simulink model "Simulator_Part_12"  (R2019b)
settings: Solver=FixedStepAuto  StartTime=0.0  StopTime=tfinal  FixedStep=dt  RelTol=1e-3
model workspace (MAT data in the model file):
  s000 = 0
values from neighbouring files (symbols this model uses):
  dc = [ aircraft_data(57:59) * pi/180 ; aircraft_data(60)]    [Aircraft_Simulator.m]    (also in Plot1.m = [da 0 0 0]; Plot2.m = [0 0 0 dT]; Plot3.m = [0 0 0 dT]; Plot4.m = [0 0 0 dT])
  Fg_0 = m*g*[sin(s0(8)); -cos(s0(8))*sin(s0(7)); -cos(s0(8))*cos(s0(7))]    [Aircraft_Simulator.m]
  g = aircraft_data(52)    [Aircraft_Simulator.m]    (also in Airframe_Model.m = 32.17405)
  Ixx = aircraft_data(53)    [Aircraft_Simulator.m]    (also in Airframe_Model.m = I(1))
  Iyy = aircraft_data(54)    [Aircraft_Simulator.m]    (also in Airframe_Model.m = I(5))
  Izz = aircraft_data(55)    [Aircraft_Simulator.m]    (also in Airframe_Model.m = I(9))
  K = struct('u',s0(1),'v',s0(2),'w',s0(3),'p',s0(4),'q',s0(5),     'r',s0(6),'phi',s0(7),'theta',s0(8),'psi',s0(9),'x',s0(10),     'y',s0(11),'z',s0(12),'alpha',s0(8),'beta',0,'V_t',Vto,'w_dot',0)    [Aircraft_Simulator.m]
  m = aircraft_data(51)    [Aircraft_Simulator.m]
  M_0 = [0; 0; 0]    [Aircraft_Simulator.m]
  Matrix_Controllers = [0     0       Xde   Xdth ... (first row only)    [Aircraft_Simulator.m]
  Matrix_states = [Xu   0   Xw   0   0   0   0 ... (first row only)    [Aircraft_Simulator.m]    (also in Airframe_Model.m)
  s0 = aircraft_data(4:15)    [Aircraft_Simulator.m]
  w_dot0 = 0    [Aircraft_Simulator.m]
libraries: dspsigops x3, shared6dof x1, aerolibasang x1
settings Model: Creator=Administrator  LastModifiedBy=Administrator

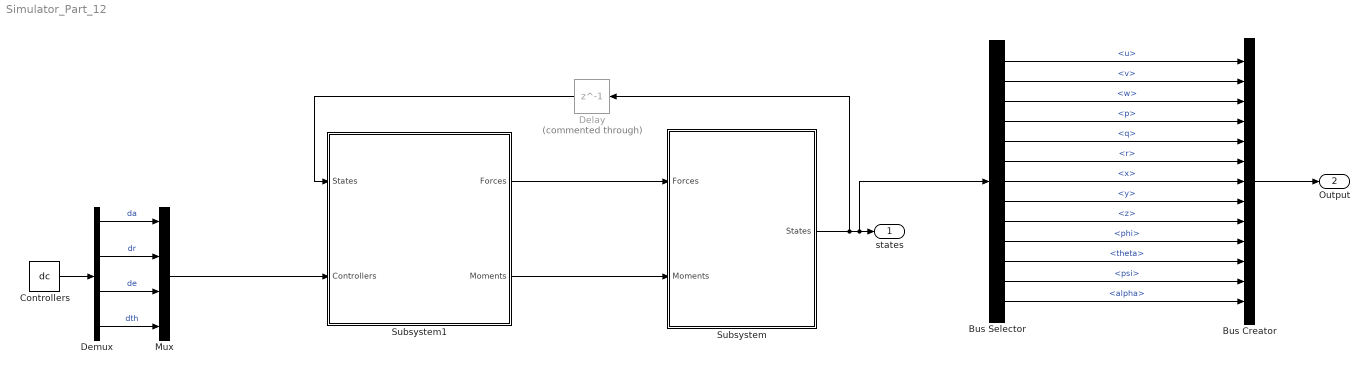
== system Simulator_Part_12 ==
  Bus Creator : BusCreator  Inputs=13
  Bus Selector : BusSelector  OutputSignals=u,v,w,p,q,r,x,y,z,phi,theta,psi,alpha
  Controllers : Constant  Value=dc
  Delay : Delay  Commented=through  DelayLength=1  InitialCondition=K
  Demux : Demux
  Mux : Mux
  Subsystem : Subsystem
  Subsystem1 : Subsystem
  states : Outport
  Output : Outport  Port=2
  wires:
  Subsystem/1(States) -> Delay/1, Bus Selector/1, states/1
  Subsystem1/1(Forces) -> Subsystem/1(Forces)
  Subsystem1/2(Moments) -> Subsystem/2(Moments)
  Delay/1 -> Subsystem1/1(States)
  Controllers/1 -> Demux/1
  Demux/3 -> Mux/3  "de"
  Demux/4 -> Mux/4  "dth"
  Demux/2 -> Mux/2  "dr"
  Demux/1 -> Mux/1  "da"
  Mux/1 -> Subsystem1/2(Controllers)
  Bus Selector/1 -> Bus Creator/1  "<u>"
  Bus Selector/2 -> Bus Creator/2  "<v>"
  Bus Selector/3 -> Bus Creator/3  "<w>"
  Bus Selector/4 -> Bus Creator/4  "<p>"
  Bus Selector/5 -> Bus Creator/5  "<q>"
  Bus Selector/6 -> Bus Creator/6  "<r>"
  Bus Selector/7 -> Bus Creator/7  "<x>"
  Bus Selector/8 -> Bus Creator/8  "<y>"
  Bus Selector/9 -> Bus Creator/9  "<z>"
  Bus Selector/10 -> Bus Creator/10  "<phi>"
  Bus Selector/11 -> Bus Creator/11  "<theta>"
  Bus Selector/12 -> Bus Creator/12  "<psi>"
  Bus Creator/1 -> Output/1
  Bus Selector/13 -> Bus Creator/13  "<alpha>"

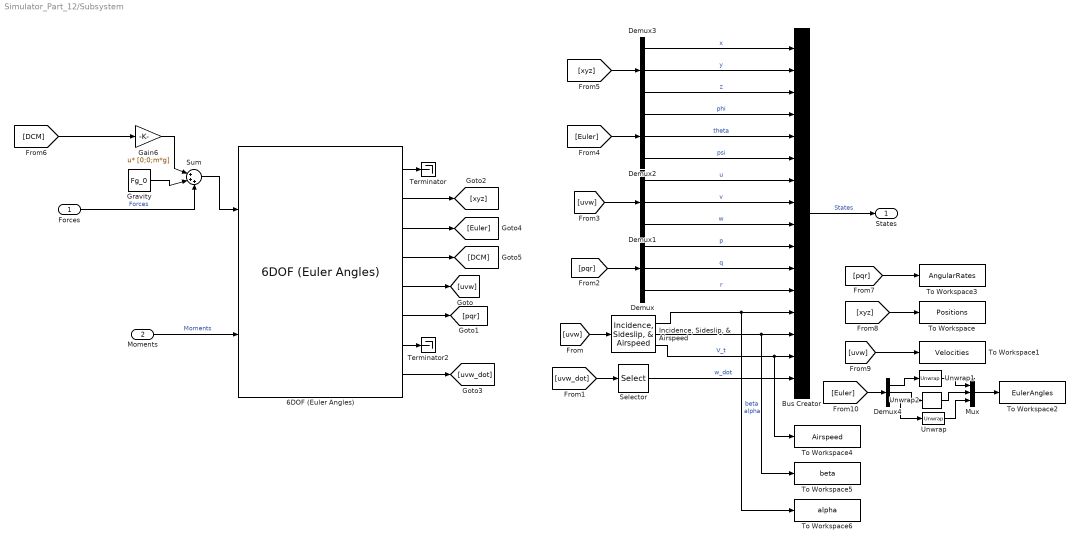
== system Simulator_Part_12/Subsystem ==
  Forces : Inport
  Moments : Inport  Port=2
  6DOF (Euler Angles) : shared6dof/6DOF (Euler Angles)  units=English (Velocity in ft/s)  mtype=Fixed  rep=Euler Angles  xme_0=s0(10:12)  Vm_0=s0(1:3)  eul_0=s0(7:9)  pm_0=s0(4:6)  mass_0=m  mass_e=0.5  mass_f=2.0  inertia=I  inertia_e=eye(3)  inertia_f=2*eye(3)  k_quat=1.0  vre_flag=on  abi_flag=off  aMode=0  xme_statename=''  Vm_statename=''  eul_statename=''  quat_statename=''  pm_statename=''  mass_statename=''
      settings: SourceProductBaseCode=AE,PW,MT,UV,VE,VP
  Bus Creator : BusCreator  Inputs=16
  Demux{,1..4} (5 alike) : Demux  Outputs=3
  Gain6 : Gain  Gain=[0;0;m*g]  Multiplication=Matrix(u*K)
  Gravity : Constant  Value=Fg_0
  "Incidence, Sideslip, & Airspeed" : aerolibasang/Incidence, Sideslip, & Airspeed
  Mux : Mux  Inputs=3
  Selector : Selector  InputPortWidth=3  IndexOptions=Index vector (dialog)  Indices=3  OutputSizes=1
  Sum : Sum  Inputs=|+++
  Terminator : Terminator
  Terminator2 : Terminator
  To Workspace : ToWorkspace  VariableName=Positions  SampleTime=-1
  To Workspace1 : ToWorkspace  VariableName=Velocities  SampleTime=-1
  To Workspace2 : ToWorkspace  VariableName=EulerAngles  SampleTime=-1
  To Workspace3 : ToWorkspace  VariableName=AngularRates  SampleTime=-1
  To Workspace4 : ToWorkspace  VariableName=Airspeed  SampleTime=-1
  To Workspace5 : ToWorkspace  VariableName=beta  SampleTime=-1
  To Workspace6 : ToWorkspace  VariableName=alpha  SampleTime=-1
  Unwrap : dspsigops/Unwrap  tol=pi  InputProcessing=Columns as channels (frame based)  running=off
  Unwrap1 : dspsigops/Unwrap  tol=pi  InputProcessing=Columns as channels (frame based)  running=off
  Unwrap2 : dspsigops/Unwrap  tol=pi  InputProcessing=Columns as channels (frame based)  running=off
  States : Outport
  wires:
  6DOF (Euler Angles)/3 -> [Euler]
  "Incidence, Sideslip, & Airspeed"/1 -> Bus Creator/13, To Workspace6/1  "alpha"
  [xyz] -> Demux3/1
  [uvw_dot] -> Selector/1
  6DOF (Euler Angles)/8 -> [uvw_dot]
  "Incidence, Sideslip, & Airspeed"/2 -> To Workspace5/1, Bus Creator/14  "beta"
  "Incidence, Sideslip, & Airspeed"/3 -> Bus Creator/15, To Workspace4/1  "V_t"
  [uvw] -> Demux1/1
  6DOF (Euler Angles)/1 -> Terminator/1
  [Euler] -> Demux2/1
  Demux/2 -> Bus Creator/11  "q"
  Bus Creator/1 -> States/1  "States"
  6DOF (Euler Angles)/7 -> Terminator2/1
  Demux1/3 -> Bus Creator/9  "w"
  Demux3/1 -> Bus Creator/1  "x"
  Demux/3 -> Bus Creator/12  "r"
  [uvw] -> "Incidence, Sideslip, & Airspeed"/1
  Demux3/3 -> Bus Creator/3  "z"
  Demux3/2 -> Bus Creator/2  "y"
  Forces/1 -> Sum/3  "Forces"
  6DOF (Euler Angles)/4 -> [DCM]
  6DOF (Euler Angles)/2 -> [xyz]
  [pqr] -> Demux/1
  Demux/1 -> Bus Creator/10  "p"
  Selector/1 -> Bus Creator/16  "w_dot"
  Demux1/2 -> Bus Creator/8  "v"
  6DOF (Euler Angles)/6 -> [pqr]
  6DOF (Euler Angles)/5 -> [uvw]
  Moments/1 -> 6DOF (Euler Angles)/2  "Moments"
  Demux1/1 -> Bus Creator/7  "u"
  Demux2/1 -> Bus Creator/4  "phi"
  Demux2/2 -> Bus Creator/5  "theta"
  Demux2/3 -> Bus Creator/6  "psi"
  Gain6/1 -> Sum/1
  Gravity/1 -> Sum/2
  [DCM] -> Gain6/1
  Sum/1 -> 6DOF (Euler Angles)/1
  [pqr] -> To Workspace3/1
  [xyz] -> To Workspace/1
  [uvw] -> To Workspace1/1
  [Euler] -> Demux4/1
  Demux4/3 -> Unwrap/1
  Unwrap/1 -> Mux/3
  Mux/1 -> To Workspace2/1
  Demux4/1 -> Unwrap1/1
  Unwrap1/1 -> Mux/1
  Demux4/2 -> Unwrap2/1
  Unwrap2/1 -> Mux/2

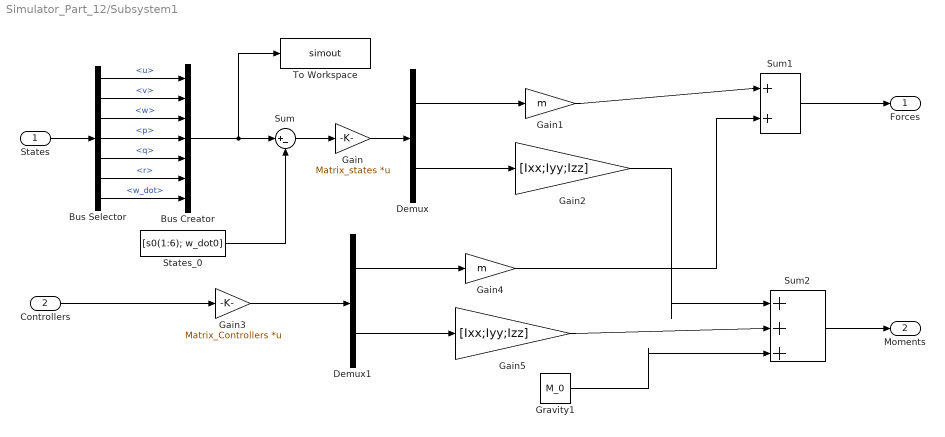
== system Simulator_Part_12/Subsystem1 ==
  States : Inport
  Controllers : Inport  Port=2
  Bus Creator : BusCreator  Inputs=7
  Bus Selector : BusSelector  OutputSignals=u,v,w,p,q,r,w_dot
  Demux : Demux  Outputs=2
  Demux1 : Demux  Outputs=2
  Gain : Gain  Gain=Matrix_states  Multiplication=Matrix(K*u)
  Gain1 : Gain  Gain=m
  Gain2 : Gain  Gain=[Ixx;Iyy;Izz]
  Gain3 : Gain  Gain=Matrix_Controllers  Multiplication=Matrix(K*u)
  Gain4 : Gain  Gain=m
  Gain5 : Gain  Gain=[Ixx;Iyy;Izz]
  Gravity1 : Constant  Value=M_0
  States_0 : Constant  Value=[s0(1:6); w_dot0]
  Sum : Sum  Inputs=|+-
  Sum1 : Sum  Inputs=|++
  Sum2 : Sum  Inputs=|+++
  To Workspace : ToWorkspace  VariableName=simout  SampleTime=-1
  Forces : Outport
  Moments : Outport  Port=2
  wires:
  Gain1/1 -> Sum1/1
  Bus Selector/6 -> Bus Creator/6  "<r>"
  Demux/2 -> Gain2/1
  Gain/1 -> Demux/1
  Gain3/1 -> Demux1/1
  Bus Selector/4 -> Bus Creator/4  "<p>"
  Sum2/1 -> Moments/1
  Sum/1 -> Gain/1
  Bus Selector/2 -> Bus Creator/2  "<v>"
  States_0/1 -> Sum/2
  Gain4/1 -> Sum1/2
  Bus Creator/1 -> To Workspace/1, Sum/1
  Bus Selector/1 -> Bus Creator/1  "<u>"
  Bus Selector/5 -> Bus Creator/5  "<q>"
  Controllers/1 -> Gain3/1
  Gravity1/1 -> Sum2/3
  Bus Selector/3 -> Bus Creator/3  "<w>"
  Bus Selector/7 -> Bus Creator/7  "<w_dot>"
  Demux/1 -> Gain1/1
  Demux1/1 -> Gain4/1
  Demux1/2 -> Gain5/1
  States/1 -> Bus Selector/1
  Gain2/1 -> Sum2/1
  Gain5/1 -> Sum2/2
  Sum1/1 -> Forces/1
